simulink model "HybridControllerPoly3_nAct"  (Simulink 6.2)
settings: Solver=FixedStepDiscrete  StartTime=0.0  StopTime=inf  FixedStep=0.001  MaxStep=.1  RelTol=1e-3
PreLoadFcn:
  | initializeSimulation
PostLoadFcn:
  | ,try, rti_mdl_postloadfcn(bdroot, 'UpdateModel', 160, 'rti1104'); catch, disp(lasterr); end,
values from neighbouring files (symbols this model uses):
  newTarget = 0    [initializeSimulation.m]
  targDsp = zeros(1,nAct)    [initializeSimulation.m]
undefined symbols (not defined in the file or in its folder): HybridCtrlParameters
libraries: rtilib1104 x3, HybridSimLib x2, simulink x2
CloseFcn:
  | rtwprivate ssgencode ModelCloseRequest HybridController2
settings Model: Creator=Andreas Schellenberg  LastModifiedBy=cwhyte  ExtModeAutoUpdateStatusClock=off  TunableVars=newTarget,targDsp  TunableVarsStorageClass=ExportedGlobal,ExportedGlobal  TunableVarsTypeQualifier=volatile,volatile  BufferReuse=off  ProdHWDeviceType=Specified
settings DataIOCC: LimitDataPoints=off  SaveOutput=off  SignalLogging=off  SaveTime=off  SignalLoggingName=sigsOut
settings OptimizationCC: BlockReduction=off  InlineParams=on  OptimizeBlockIOStorage=off  BufferReuse=off  EnforceIntegerDowncast=off  ExpressionFolding=off  FoldNonRolledExpr=off  LocalBlockOutputs=off  StateBitsets=on  DataBitsets=on  UseTempVars=on
settings DebuggingCC: SignalResolutionControl=UseLocalSettings
settings HardwareCC: ProdIntDivRoundTo=Zero  ProdEndianess=BigEndian  ProdHWDeviceType=Specified  TargetIntDivRoundTo=Zero  TargetEndianess=BigEndian
settings RTWCC: SystemTargetFile=rti1104.tlc  MakeCommand=make_rti  TemplateMakefile=rti1104.tmf  Description=dSPACE DS1104 Hardware Platform  ProcessScript=rti1104_make_rtw_hook  CustomHeaderCode="#include \"PredictorCorrector.h\""  CustomSource=PredictorCorrector.c
settings STFCustomTargetCC: TargetFcnLib=ansi_tfl_tmw.mat  GenFloatMathFcnCalls=ANSI_C  ModelReferenceCompliant=off  LogVarNameModifier=none  MatFileLogging=on  SystemTargetFile=rti1104.tlc
settings GRTTargetCC: ModelReferenceCompliant=off  LogVarNameModifier=none  ExtModeMexFile=rti_comm
settings CustomProperty: DataType=RTWOptions_EnumType_c__dspace_matlab_rti1104_tlc_rti1104_InitialSimState  Value=STOP
settings EnumStrPairs: String=RUN

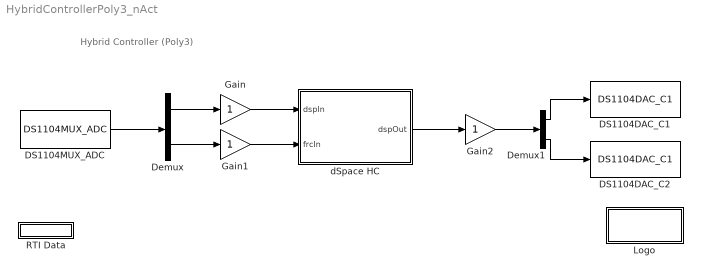
== system HybridControllerPoly3_nAct ==
  note: Hybrid Controller (Poly3)
  DS1104DAC_C1 : rtilib1104/DS1104 MASTER PPC/DS1104DAC_C1  ChannelNo=1  InitValue=0  TermMode=0  TermValue=0  Reserved1=[]  Reserved2=[]  Reserved3=[]  Reserved4=[]  DialogFcn=gui1104dac  UnitName={ 'DS1104DAC_C'}  UnitValues={ 1 }  DSProperties=struct('RTI',struct('Version',uint32(1),'BlockType',struct('isSLSource',uint8(0),'isSLSink',uint8(1),'isHWSource',uint8(0),'isHWSink',uint8(1),'isSetup',uint8(0),'isInline',uint8(1),'isNonInline',uint8(0),'isInterrupt',uint8(0),'isChannelwise',uint8(1)),'IOBoardType','DS1104MASTER','UnitType','DAC','Identifier','DAC','DialogType','ML','BlockSet','NONE','SlaveProcessor','NONE'))
  DS1104DAC_C2 : rtilib1104/DS1104 MASTER PPC/DS1104DAC_C1  ChannelNo=2  InitValue=0  TermMode=0  TermValue=0  Reserved1=[]  Reserved2=[]  Reserved3=[]  Reserved4=[]  DialogFcn=gui1104dac  UnitName={ 'DS1104DAC_C'}  UnitValues={2}  DSProperties=struct('RTI',struct('Version',uint32(1),'BlockType',struct('isSLSource',uint8(0),'isSLSink',uint8(1),'isHWSource',uint8(0),'isHWSink',uint8(1),'isSetup',uint8(0),'isInline',uint8(1),'isNonInline',uint8(0),'isInterrupt',uint8(0),'isChannelwise',uint8(1)),'IOBoardType','DS1104MASTER','UnitType','DAC','Identifier','DAC','DialogType','ML','BlockSet','NONE','SlaveProcessor','NONE'))
  DS1104MUX_ADC : rtilib1104/DS1104 MASTER PPC/DS1104MUX_ADC  ChannelNos=[1 2 3 4]  TriggerMode=0  Reserved1=[]  Reserved2=[]  Reserved3=[]  Reserved4=[]  DialogFcn=gui1104mux_adc  UnitName={ 'DS1104MUX_ADC' }  UnitValues={ [] }  DSProperties=struct('RTI',struct('Version',uint32(1),'BlockType',struct('isSLSource',uint8(1),'isSLSink',uint8(0),'isHWSource',uint8(1),'isHWSink',uint8(0),'isSetup',uint8(0),'isInline',uint8(1),'isNonInline',uint8(0),'isInterrupt',uint8(0),'isChannelwise',uint8(0)),'IOBoardType','DS1104MASTER','UnitType','ADC','Identifier','ADCMUX','DialogType','ML','BlockSet','NONE','SlaveProcessor','NONE'))
  Demux : Demux  Outputs=2
  Demux1 : Demux  Outputs=2
  Gain : Gain  SaturateOnIntegerOverflow=on
  Gain1 : Gain  SaturateOnIntegerOverflow=on
  Gain2 : Gain  SaturateOnIntegerOverflow=on
  Logo : Subsystem  mask(dSPACE){EmptyParameter=}
      mask prompts: EmptyParameter "Mask Parameter 1:"
      settings: OpenFcn=;
      mask Display: image(imread('rti_mdl_dslogo.tif'));
  RTI Data : Subsystem  Tag=struct('RTIDataServer',struct('RTIDataServerVs','2','RTIModelDescription','struct(''main'',''HybridControllerPoly3_nAct'',''sub'','''',''isMp'',0)'))  LoadFcn="if exist('rtidc'), try,  rtidc('DataHostBlockClbLoad', gcbh); catch, disp(['Warning: ''LoadFcn'' for RTI Data block failed: ' lasterr]); end, end,"
      settings: CopyFcn="if exist('rtidc'), try,  rtidc('DataHostBlockClbCopy', gcbh); catch, disp(['Warning: ''CopyFcn'' for RTI Data block failed: ' lasterr]); end, end,"  DeleteFcn="if exist('rtidc'), try,  rtidc('DataHostBlockClbDelete', gcbh); catch, disp(['Warning: ''DeleteFcn'' for RTI Data block failed: ' lasterr]); end, end,"  ModelCloseFcn="if exist('rtidc'), try,  rtidc('DataHostBlockClbModelClose', gcbh); catch, disp(['Warning: ''ModelCloseFcn'' for RTI Data block failed: ' lasterr]); end, end,"  PreSaveFcn="if exist('rtidc'), try,  rtidc('DataHostBlockClbPreSave', gcbh); catch, disp(['Warning: ''PreSaveFcn'' for RTI Data block failed: ' lasterr]); end, end,"  PostSaveFcn="if exist('rtidc'), try,  rtidc('DataHostBlockClbPostSave', gcbh); catch, disp(['Warning: ''PostSaveFcn'' for RTI Data block failed: ' lasterr]); end, end,"  NameChangeFcn="if exist('rtidc'), try,  rtidc('DataHostBlockClbNameChange', gcbh); catch, disp(['Warning: ''NameChangeFcn'' for RTI Data block failed: ' lasterr]); end, end,"
      mask Type: RTI_DATA_HOST
      mask Description:
      | RTI Data Block.
      | This block is used by RTI to store internal model-dependent data.
      | Please keep this block on the root level of the model. Deleting this block will result in data loss.
      | 
      | NEVER DELETE OR COPY THIS BLOCK!
      mask Help:
      | RTI Data Block.
      | This block is used by RTI to store internal model-dependent data.
      | Please keep this block on the root level of the model. Deleting this block will result in data loss.
      | 
      | NEVER DELETE OR COPY THIS BLOCK!
      mask Display:
      | text(0.5, 0.5, 'RTI Data', 'HorizontalAlignment', 'center');
      | plot([1 0]);
  dSpace HC : Subsystem  AncestorBlock=HybridSimLib/xPC Target/xPC HC1  mask(Hybrid Controller: Poly3){nAct=2, dtInt=HybridCtrlParameters.dtInt, dtSim=HybridCtrlParameters.dtSim, dtCon=HybridCtrlParameters.dtCon, N=HybridCtrlParameters.N, iDelay=HybridCtrlParameters.iDelay, dspLim=HybridCtrlParameters.dspLim, velLim=HybridCtrlParameters.velLim}
      mask prompts: nAct "Number of Actuators: nAct"; dtInt "Integration time step: dtInt"; dtSim "Simulation time step: dtSim"; dtCon "Controller time step: dtCon"; N "Maximum number of substeps: N"; iDelay "Number of delay steps: iDelay"; dspLim "Displacement limit: dspLim"; velLim "Velocity limit: velLim"
      mask help: Hybrid Controller using cubic Lagrange interpolation for prediction and correction
      mask Display: disp('dSpace\nHybrid Controller\n(Poly3)')
  wires:
  dSpace HC/1(dspOut) -> Gain2/1
  Gain/1 -> dSpace HC/1(dspIn)
  Gain1/1 -> dSpace HC/2(frcIn)
  DS1104MUX_ADC/1 -> Demux/1
  Demux/1 -> Gain/1
  Demux/2 -> Gain1/1
  Gain2/1 -> Demux1/1
  Demux1/2 -> DS1104DAC_C2/1
  Demux1/1 -> DS1104DAC_C1/1

== system HybridControllerPoly3_nAct/Logo ==
  note: $Workfile: demo1104_analog.mdl $
  note: $Date: 15.05.01 13:54 $
  note: $Revision: 3 $

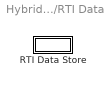
== system HybridControllerPoly3_nAct/RTI Data ==
  RTI Data Store : Subsystem  Tag="struct('private',struct('version',struct('dsVer',uint32(2),'dsVerCreation',uint32(2),'RTI',struct('ver','4.1a3','type','RTI1104')),'access',struct('type','Model','isPerm',1,'created',['13-Feb-2001 14:58:17'],'modified',['18-Oct-2007 18:15:22'],'location','')),'public',struct('main',struct('data',[]),'sub',struct('name',{{'HybridControllerPoly3_nAct'}},'data',{{struct('TH',struct('thTaskInfo',struct('taskType',{'TIMER','HWINT','TMRINT','SWINT'},'tasksNumOf',{1,0,0,0},'srcIds',{{'TIMERA'},{},{},{}},'taskNames',{{['Timer Task 1']},{},{},{}})),'th_tc',struct('dataType','TASK','taskGroupId','','taskGroupList',{{}},'taskSchedulingPolicy','FCFS','taskType','TIMER','blkh',-1,'srcId','TIMERA','srcSgnName',['Timer A interrupt'],'srcCpuName','','taskName',['Timer Task 1  [0.001] s'],'taskNameDisplayExt','','smplTime',0.001,'smplTimeOffs',0,'hasFixedPriority',0,'priority',1,'hasFixedOvc',0,'ovcType',1,'ovcMax',0),'tc_th',struct('dataType','TASK','taskGroupId','','taskGroupList',{{}},'taskSchedulingPolicy','FCFS','taskType','TIMER','blkh',-1,'srcId','TIMERA','srcSgnName',['Timer A interrupt'],'srcCpuName','','taskName',['Timer Task 1  [0.001] s'],'taskNameDisplayExt','','smplTime',0.001,'smplTimeOffs',0,'hasFixedPriority',0,'priority',1,'hasFixedOvc',0,'ovcType',1,'ovcMax',0))}})))"
      mask Type: RTI_DATA_STORE
      mask Description:
      | RTI Data Store Block. This block is used by RTI to store internal model dependent data. Deleting this block will result in data loss.
      | 
      | NEVER DELETE, COPY, OR MODIFY THIS BLOCK!
      mask Help:
      | RTI Data Store Block. This block is used by RTI to store internal model dependent data. Deleting this block will result in data loss.
      | 
      | NEVER DELETE, COPY, OR MODIFY THIS BLOCK!
      mask Display: text(0.5, 0.5, ' ', 'HorizontalAlignment', 'center');

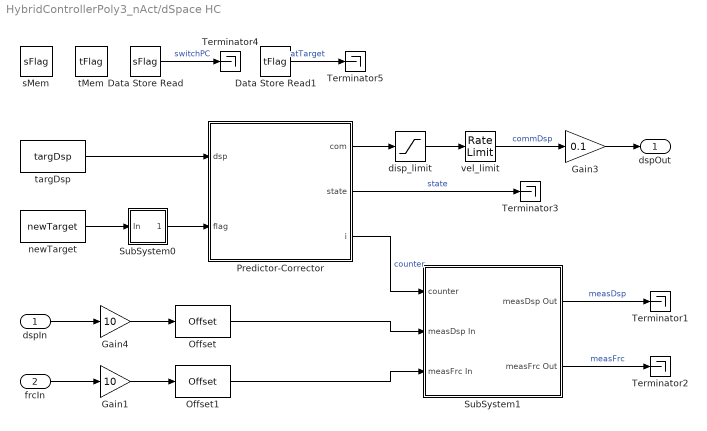
== system HybridControllerPoly3_nAct/dSpace HC ==
  dspIn : Inport  Port=1  LatchInput=off
  frcIn : Inport  Port=2  LatchInput=off
  Data Store Read : DataStoreRead  DataStoreName=sFlag  SampleTime=dtCon
  Data Store Read1 : DataStoreRead  DataStoreName=tFlag  SampleTime=dtCon
  Gain1 : Gain  Gain=10  SaturateOnIntegerOverflow=on
  Gain3 : Gain  Gain=0.1  SaturateOnIntegerOverflow=on
  Gain4 : Gain  Gain=10  SaturateOnIntegerOverflow=on
  Offset : HybridSimLib/Signal Routing/Offset  nS=nAct  nOffset=1024  dt=dtCon
  Offset1 : HybridSimLib/Signal Routing/Offset  nS=nAct  nOffset=1024  dt=dtCon
  Predictor-Corrector : Stateflow chart
  SubSystem0 : Subsystem
  SubSystem1 : Subsystem
  Terminator{1..5} (5 alike) : Terminator
  disp_limit : Saturate  UpperLimit=dspLim  LowerLimit=-dspLim
  newTarget : Constant  Value=newTarget  OutDataTypeMode=uint32  SampleTime=dtCon
  sMem : DataStoreMemory  DataStoreName=sFlag  InitialValue=0  DataType=uint32
  tMem : DataStoreMemory  DataStoreName=tFlag  InitialValue=0  DataType=uint32
  targDsp : Constant  Value=targDsp  SampleTime=dtCon
  vel_limit : RateLimiter  RisingSlewLimit=velLim  FallingSlewLimit=-velLim
  dspOut : Outport
  wires:
  frcIn/1 -> Gain1/1
  dspIn/1 -> Gain4/1
  SubSystem1/2(measFrc Out) -> Terminator2/1  "measFrc"
  SubSystem1/1(measDsp Out) -> Terminator1/1  "measDsp"
  Predictor-Corrector/3(i) -> SubSystem1/1(counter)  "counter"
  Predictor-Corrector/2(state) -> Terminator3/1  "state"
  Offset/1 -> SubSystem1/2(measDsp In)
  SubSystem0/1(Out) -> Predictor-Corrector/2(flag)
  newTarget/1 -> SubSystem0/1(In)
  targDsp/1 -> Predictor-Corrector/1(dsp)
  Offset1/1 -> SubSystem1/3(measFrc In)
  disp_limit/1 -> vel_limit/1
  vel_limit/1 -> Gain3/1  "commDsp"
  Predictor-Corrector/1(com) -> disp_limit/1
  Gain3/1 -> dspOut/1
  Gain4/1 -> Offset/1
  Gain1/1 -> Offset1/1
  Data Store Read/1 -> Terminator4/1  "switchPC"
  Data Store Read1/1 -> Terminator5/1  "atTarget"

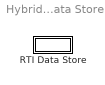
== system HybridControllerPoly3_nAct/RTI Data/RTI Data Store ==
  RTI Data Store : Subsystem
      mask Type: RTI_DATA_STORE
      mask Description:
      | RTI Data Store Block. This block is used by RTI to store internal model dependent data. Deleting this block will result in data loss.
      | 
      | NEVER DELETE, COPY, OR MODIFY THIS BLOCK!
      mask Help:
      | RTI Data Store Block. This block is used by RTI to store internal model dependent data. Deleting this block will result in data loss.
      | 
      | NEVER DELETE, COPY, OR MODIFY THIS BLOCK!
      mask Display: text(0.5, 0.5, ' ', 'HorizontalAlignment', 'center');

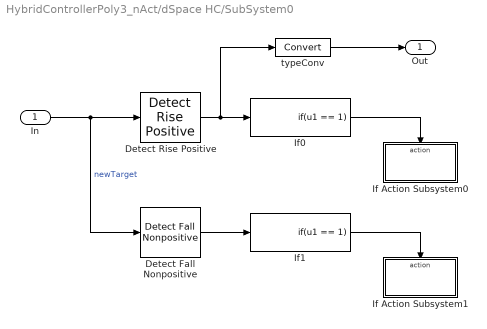
== system HybridControllerPoly3_nAct/dSpace HC/SubSystem0 ==
  In : Inport  Port=1  LatchInput=off
  Detect Fall Nonpositive : simulink/Logic and Bit Operations/Detect Fall Nonpositive  vinit=0
  Detect Rise Positive : simulink/Logic and Bit Operations/Detect Rise Positive  vinit=0
  If Action Subsystem0 : Subsystem  TreatAsAtomicUnit=on
  If Action Subsystem1 : Subsystem  TreatAsAtomicUnit=on
  If0 : If  IfExpression=u1 == 1  ShowElse=off
  If1 : If  IfExpression=u1 == 1  ShowElse=off
  typeConv : DataTypeConversion  OutDataTypeMode=uint32  SaturateOnIntegerOverflow=on  RndMeth=Zero
  Out : Outport
  wires:
  In/1 -> Detect Rise Positive/1, Detect Fall Nonpositive/1  "newTarget"
  Detect Rise Positive/1 -> If0/1, typeConv/1
  Detect Fall Nonpositive/1 -> If1/1
  If1/1 -> If Action Subsystem1/Action
  If0/1 -> If Action Subsystem0/Action
  typeConv/1 -> Out/1

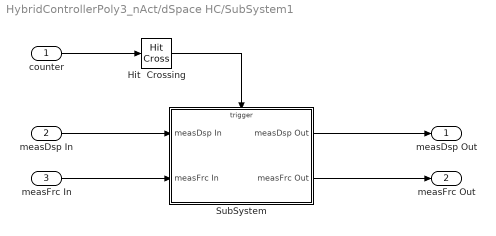
== system HybridControllerPoly3_nAct/dSpace HC/SubSystem1 ==
  counter : Inport  Port=1  LatchInput=off
  measDsp In : Inport  Port=2  LatchInput=off
  measFrc In : Inport  Port=3  LatchInput=off
  Hit  Crossing : HitCross  HitCrossingOffset=iDelay
  SubSystem : Subsystem  TreatAsAtomicUnit=on
  measDsp Out : Outport
  measFrc Out : Outport  Port=2
  wires:
  SubSystem/2(measFrc Out) -> measFrc Out/1
  measFrc In/1 -> SubSystem/2(measFrc In)
  SubSystem/1(measDsp Out) -> measDsp Out/1
  measDsp In/1 -> SubSystem/1(measDsp In)
  counter/1 -> Hit  Crossing/1
  Hit  Crossing/1 -> SubSystem/Trigger

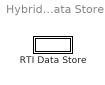
== system HybridControllerPoly3_nAct/RTI Data/RTI Data Store/RTI Data Store ==
  RTI Data Store : Subsystem
      mask Type: RTI_DATA_STORE
      mask Description:
      | RTI Data Store Block. This block is used by RTI to store internal model dependent data. Deleting this block will result in data loss.
      | 
      | NEVER DELETE, COPY, OR MODIFY THIS BLOCK!
      mask Help:
      | RTI Data Store Block. This block is used by RTI to store internal model dependent data. Deleting this block will result in data loss.
      | 
      | NEVER DELETE, COPY, OR MODIFY THIS BLOCK!
      mask Display: text(0.5, 0.5, ' ', 'HorizontalAlignment', 'center');

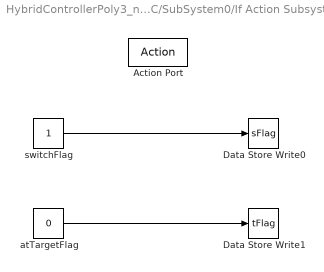
== system HybridControllerPoly3_nAct/dSpace HC/SubSystem0/If Action Subsystem0 ==
  Action Port : ActionPort  ActionType=then
  Data Store Write0 : DataStoreWrite  DataStoreName=sFlag  SampleTime=-1
  Data Store Write1 : DataStoreWrite  DataStoreName=tFlag  SampleTime=-1
  atTargetFlag : Constant  Value=0  OutDataTypeMode=uint32  SampleTime=dtCon
  switchFlag : Constant  OutDataTypeMode=uint32  SampleTime=dtCon
  wires:
  atTargetFlag/1 -> Data Store Write1/1
  switchFlag/1 -> Data Store Write0/1

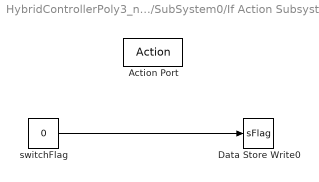
== system HybridControllerPoly3_nAct/dSpace HC/SubSystem0/If Action Subsystem1 ==
  Action Port : ActionPort  ActionType=then
  Data Store Write0 : DataStoreWrite  DataStoreName=sFlag  SampleTime=-1
  switchFlag : Constant  Value=0  OutDataTypeMode=uint32  SampleTime=dtCon
  wires:
  switchFlag/1 -> Data Store Write0/1

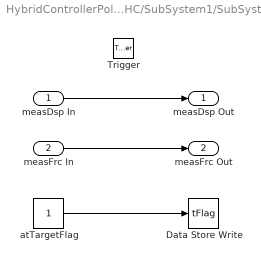
== system HybridControllerPoly3_nAct/dSpace HC/SubSystem1/SubSystem ==
  measDsp In : Inport  Port=1  LatchInput=off
  measFrc In : Inport  Port=2  LatchInput=off
  Trigger : TriggerPort
  Data Store Write : DataStoreWrite  DataStoreName=tFlag  SampleTime=-1
  atTargetFlag : Constant  OutDataTypeMode=uint32  SampleTime=-1
  measDsp Out : Outport  InitialOutput=[0]
  measFrc Out : Outport  Port=2  InitialOutput=[0]
  wires:
  atTargetFlag/1 -> Data Store Write/1
  measFrc In/1 -> measFrc Out/1
  measDsp In/1 -> measDsp Out/1

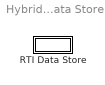
== system HybridControllerPoly3_nAct/RTI Data/RTI Data Store/RTI Data Store/RTI Data Store ==
  RTI Data Store : Subsystem
      mask Type: RTI_DATA_STORE
      mask Description:
      | RTI Data Store Block. This block is used by RTI to store internal model dependent data. Deleting this block will result in data loss.
      | 
      | NEVER DELETE, COPY, OR MODIFY THIS BLOCK!
      mask Help:
      | RTI Data Store Block. This block is used by RTI to store internal model dependent data. Deleting this block will result in data loss.
      | 
      | NEVER DELETE, COPY, OR MODIFY THIS BLOCK!
      mask Display: text(0.5, 0.5, ' ', 'HorizontalAlignment', 'center');

== system HybridControllerPoly3_nAct/RTI Data/RTI Data Store/RTI Data Store/RTI Data Store/RTI Data Store ==

== stateflow chart dSpace HC/Predictor-Corrector ==
  state HybridController [parallel]
    state Predict
      en: state = 1;
      en: diSD = 1;
      en: i = 1; iSD = 0;
      en: predictP3(com,i/N);
      du: i++;
      du: predictP3(com,i/N);
    state Initialize
      en: i = 1; iSD = 0;
      en: diSD = 1;
      en: initData(nAct,dtCon);
      en: zeroDsp(com);
    state AutoSlowDown
      en: state = 2;
      en: diSD = 4-i/(0.2*N);
      en: i += diSD; iSD = i;
      en: predictP3(com,i/N);
      du: diSD = 4-i/(0.2*N);
      du: i += diSD; iSD = i;
      du: predictP3(com,i/N);
    state Correct
      en: state = 0;
      en: setCurDsp(com,i/N);
      en: dspLocal = dsp; setNewDsp(dspLocal);
      en: di = min(max(diSD+1/(0.2*N)*(i-iSD),0.001),1.0);
      en: i = min(i+di,N);
      en: correctP3(com,i/N);
      du: di = min(max(diSD+1/(0.2*N)*(i-iSD),0.001),1.0);
      du: i = min(i+di,N);
      du: correctP3(com,i/N);
    Correct -> Predict : [i>=N]
    (default) -> Initialize
    Predict -> Correct [order 2] : [flag==1]
    Initialize -> Correct : [flag==1]
    AutoSlowDown -> Correct : [flag==1]
    Predict -> AutoSlowDown [order 1] : [i>=0.6*N && flag~=1]
  data: dsp input double size=nAct; flag input uint32; com output double size=nAct; state output uint32; i output double; N local double; nAct parameter uint32 =1; iDelay local double; di local double; diSD local double; iSD local double; dspLocal local double size=nAct
